simulink model "gm_mandelbrot_fpga"  (R2019b)
settings: Solver=FixedStepDiscrete  StartTime=0.0  StopTime=33.5e-3  FixedStep=0.5*Ts  RelTol=1e-3  EnableMultiTasking=on
undefined symbols (not defined in the file or in its folder): BUTTON_CLOCK_DIV, BUTTON_DEBOUNCE, BUTTON_POLLING, LUT_BLUE, LUT_GREEN, LUT_RED, MAX_ITERATIONS, PIXEL_TIME, TRASLATION_FACTOR, Ts, VGA_HORIZONTAL_BACK_PORCH, VGA_HORIZONTAL_FRONT_PORCH, VGA_HORIZONTAL_RESOLUTION, VGA_HORIZONTAL_SYNC, VGA_VERTICAL_BACK_PORCH, VGA_VERTICAL_FRONT_PORCH, VGA_VERTICAL_RESOLUTION, VGA_VERTICAL_SYNC, ZOOM_FACTOR
libraries: simulink x132, hdlsllib x20, visionsinks x1
(part 3 of 9)

== system gm_mandelbrot_fpga/mandelbrot_top/mandelbrot_core/plane_converter  ==
  zoom : Inport  OutDataTypeStr=fixdt(1, 18, 15)  PortDimensions=1  SampleTime=1.35e-08
  "horizontal_offset " : Inport  Port=2  OutDataTypeStr=fixdt(1, 18, 15)  PortDimensions=1  SampleTime=1.35e-08
  "vertical_offset " : Inport  Port=3  OutDataTypeStr=fixdt(1, 18, 15)  PortDimensions=1  SampleTime=1.35e-08
  "horizontal_index " : Inport  Port=4  OutDataTypeStr=uint16  PortDimensions=1  SampleTime=1.35e-08
  "vertical_index " : Inport  Port=5  OutDataTypeStr=uint16  PortDimensions=1  SampleTime=1.35e-08
  Add : Sum
  Add1 : Sum
  Constant1 : Constant  Value=VGA_VERTICAL_RESOLUTION/2.0  OutDataTypeStr=fixdt(1,12,0)  SampleTime=-1
  Constant2 : Constant  Value=2.0/VGA_VERTICAL_RESOLUTION  OutDataTypeStr=Z_BUS_TYPE  SampleTime=-1
  Constant4 : Constant  Value=VGA_HORIZONTAL_RESOLUTION/2.0  OutDataTypeStr=fixdt(1,12,0)  SampleTime=-1
  Data Type Conversion : DataTypeConversion
  Data Type Conversion1 : DataTypeConversion
  Data Type Conversion2 : DataTypeConversion
  Product1 : Product
  Product2 : Product
  Product3 : Product
  Real-Imag to Complex : RealImagToComplex
  Subtract : Sum  Inputs=-+
  Subtract1 : Sum  Inputs=+-
  Unit Delay : UnitDelay  SampleTime=-1  HasFrameUpgradeWarning=on
  c : Outport  OutDataTypeStr=Z_BUS_TYPE  VectorParamsAs1DForOutWhenUnconnected=off
  wires:
  zoom/1 -> Product1/1
  "horizontal_offset "/1 -> Add/1
  "vertical_offset "/1 -> Add1/1
  "horizontal_index "/1 -> Data Type Conversion/1
  "vertical_index "/1 -> Data Type Conversion1/1
  Add/1 -> Real-Imag to Complex/1
  Add1/1 -> Real-Imag to Complex/2
  Constant1/1 -> Subtract1/1
  Constant2/1 -> Product3/2, Product2/2
  Constant4/1 -> Subtract/1
  Data Type Conversion/1 -> Subtract/2
  Data Type Conversion1/1 -> Subtract1/2
  Data Type Conversion2/1 -> c/1
  Product1/1 -> Data Type Conversion2/1
  Product2/1 -> Add/2
  Product3/1 -> Add1/2
  Real-Imag to Complex/1 -> Unit Delay/1
  Subtract/1 -> Product2/1
  Subtract1/1 -> Product3/1
  Unit Delay/1 -> Product1/2

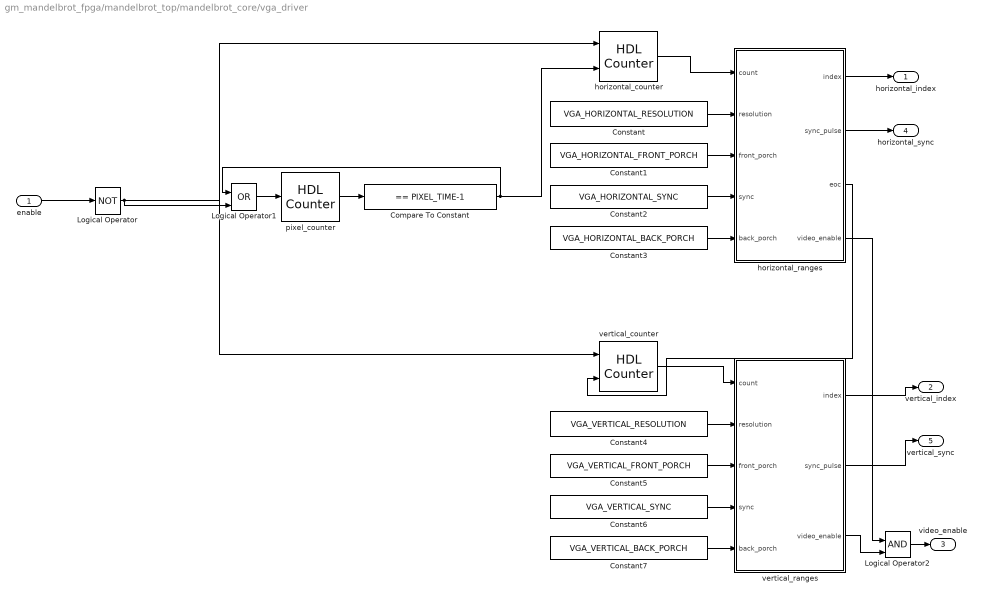
== system gm_mandelbrot_fpga/mandelbrot_top/mandelbrot_core/vga_driver ==
  "enable " : Inport  OutDataTypeStr=boolean  PortDimensions=1  SampleTime=1.35e-08
  Compare To Constant : simulink/Logic and Bit Operations/Compare To Constant  relop===  const=PIXEL_TIME-1  OutDataTypeStr=boolean
  Constant : Constant  Value=VGA_HORIZONTAL_RESOLUTION  OutDataTypeStr=uint16  SampleTime=-1
  Constant1 : Constant  Value=VGA_HORIZONTAL_FRONT_PORCH  OutDataTypeStr=uint16  SampleTime=-1
  Constant2 : Constant  Value=VGA_HORIZONTAL_SYNC  OutDataTypeStr=uint16  SampleTime=-1
  Constant3 : Constant  Value=VGA_HORIZONTAL_BACK_PORCH  OutDataTypeStr=uint16  SampleTime=-1
  Constant4 : Constant  Value=VGA_VERTICAL_RESOLUTION  OutDataTypeStr=uint16  SampleTime=-1
  Constant5 : Constant  Value=VGA_VERTICAL_FRONT_PORCH  OutDataTypeStr=uint16  SampleTime=-1
  Constant6 : Constant  Value=VGA_VERTICAL_SYNC  OutDataTypeStr=uint16  SampleTime=-1
  Constant7 : Constant  Value=VGA_VERTICAL_BACK_PORCH  OutDataTypeStr=uint16  SampleTime=-1
  Logical Operator : Logic  Operator=NOT  IconShape=distinctive  AllPortsSameDT=off  OutDataTypeStr=boolean
  Logical Operator1 : Logic  Operator=OR  IconShape=distinctive  AllPortsSameDT=off  OutDataTypeStr=boolean
  Logical Operator2 : Logic  IconShape=distinctive  AllPortsSameDT=off  OutDataTypeStr=boolean
  horizontal_counter : hdlsllib/Sources/HDL Counter  CountType=Count limited  CountInit=0  CountStep=1  CountMax=VGA_HORIZONTAL_RESOLUTION+VGA_HORIZONTAL_FRONT_PORCH+VGA_HORIZONTAL_SYNC+VGA_HORIZONTAL_BACK_PORCH-1  CountFromType=Initial value  CountFrom=0  CountResetPort=on  CountLoadPort=off  CountEnbPort=on  CountDirPort=off  CountDataType=Unsigned  CountWordLen=16  CountFracLen=0  CountSampTime=1
      settings: SourceProductName=Simulink
  horizontal_ranges : Subsystem
  "pixel_counter " : hdlsllib/Sources/HDL Counter  CountType=Count limited  CountInit=0  CountStep=1  CountMax=PIXEL_TIME  CountFromType=Initial value  CountFrom=0  CountResetPort=on  CountLoadPort=off  CountEnbPort=off  CountDirPort=off  CountDataType=Unsigned  CountWordLen=8  CountFracLen=0  CountSampTime=Ts
      settings: SourceProductName=Simulink
  "vertical_counter " : hdlsllib/Sources/HDL Counter  CountType=Count limited  CountInit=0  CountStep=1  CountMax=VGA_VERTICAL_RESOLUTION+VGA_VERTICAL_FRONT_PORCH+VGA_VERTICAL_SYNC+VGA_VERTICAL_BACK_PORCH-1  CountFromType=Initial value  CountFrom=0  CountResetPort=on  CountLoadPort=off  CountEnbPort=on  CountDirPort=off  CountDataType=Unsigned  CountWordLen=16  CountFracLen=0  CountSampTime=1
      settings: SourceProductName=Simulink
  "vertical_ranges " : Subsystem
  horizontal_index : Outport  VectorParamsAs1DForOutWhenUnconnected=off
  vertical_index : Outport  Port=2  VectorParamsAs1DForOutWhenUnconnected=off
  "video_enable " : Outport  Port=3  OutDataTypeStr=boolean  VectorParamsAs1DForOutWhenUnconnected=off
  horizontal_sync : Outport  Port=4  OutDataTypeStr=boolean  VectorParamsAs1DForOutWhenUnconnected=off
  "vertical_sync " : Outport  Port=5  OutDataTypeStr=boolean  VectorParamsAs1DForOutWhenUnconnected=off
  wires:
  "enable "/1 -> Logical Operator/1
  Compare To Constant/1 -> Logical Operator1/1, horizontal_counter/2
  Constant/1 -> horizontal_ranges/2(resolution)
  Constant1/1 -> horizontal_ranges/3(front_porch)
  Constant2/1 -> horizontal_ranges/4("sync ")
  Constant3/1 -> horizontal_ranges/5(back_porch)
  Constant4/1 -> "vertical_ranges "/2(resolution)
  Constant5/1 -> "vertical_ranges "/3(front_porch)
  Constant6/1 -> "vertical_ranges "/4("sync ")
  Constant7/1 -> "vertical_ranges "/5(back_porch)
  Logical Operator/1 -> Logical Operator1/2, "vertical_counter "/1, horizontal_counter/1
  Logical Operator1/1 -> "pixel_counter "/1
  Logical Operator2/1 -> "video_enable "/1
  horizontal_counter/1 -> horizontal_ranges/1("count ")
  horizontal_ranges/1("index ") -> horizontal_index/1
  horizontal_ranges/2("sync_pulse ") -> horizontal_sync/1
  horizontal_ranges/3("eoc ") -> "vertical_counter "/2
  horizontal_ranges/4(video_enable) -> Logical Operator2/1
  "pixel_counter "/1 -> Compare To Constant/1
  "vertical_counter "/1 -> "vertical_ranges "/1("count ")
  "vertical_ranges "/1("index ") -> vertical_index/1
  "vertical_ranges "/2("sync_pulse ") -> "vertical_sync "/1
  "vertical_ranges "/3(video_enable) -> Logical Operator2/2

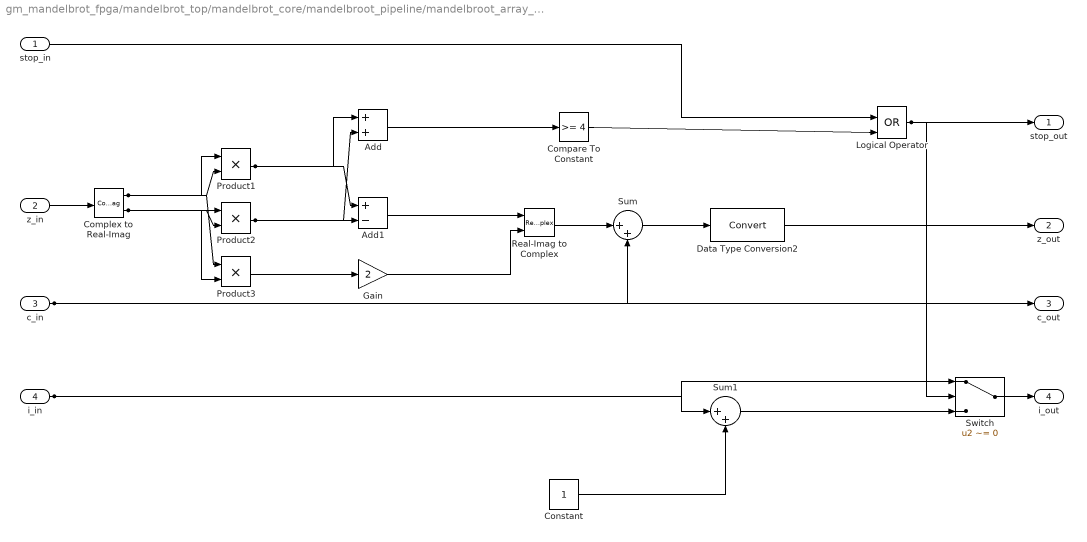
== system gm_mandelbrot_fpga/mandelbrot_top/mandelbrot_core/mandelbroot_pipeline/mandelbroot_array_instance1 ==
  stop_in : Inport  OutDataTypeStr=boolean  PortDimensions=1  SampleTime=1.35e-08
  z_in : Inport  Port=2  OutDataTypeStr=fixdt(1, 18, 15)  PortDimensions=1  SampleTime=1.35e-08
      settings: SignalType=complex
  c_in : Inport  Port=3  OutDataTypeStr=fixdt(1, 18, 15)  PortDimensions=1  SampleTime=1.35e-08
      settings: SignalType=complex
  i_in : Inport  Port=4  OutDataTypeStr=fixdt(0, 7, 0)  PortDimensions=1  SampleTime=1.35e-08
  Add : Sum
  Add1 : Sum  Inputs=+-  OutDataTypeStr=Inherit: Same as first input
  Compare To Constant : simulink/Logic and Bit Operations/Compare To Constant  relop=>=  const=4  OutDataTypeStr=boolean
  Complex to Real-Imag : ComplexToRealImag
  Constant : Constant  OutDataTypeStr=uint8  SampleTime=-1
  Data Type Conversion2 : DataTypeConversion
  Gain : Gain  Gain=2  OutDataTypeStr=Inherit: Same as input  ParamDataTypeStr=Inherit: Same as input
  Logical Operator : Logic  Operator=OR  IconShape=distinctive  AllPortsSameDT=off  OutDataTypeStr=boolean
  Product1 : Product
  Product2 : Product
  Product3 : Product
  Real-Imag to Complex : RealImagToComplex
  Sum : Sum  Inputs=|++  OutDataTypeStr=Inherit: Same as first input
  Sum1 : Sum  Inputs=|++
  Switch : Switch  Criteria=u2 ~= 0
  stop_out : Outport  VectorParamsAs1DForOutWhenUnconnected=off
  z_out : Outport  Port=2  VectorParamsAs1DForOutWhenUnconnected=off
  c_out : Outport  Port=3  VectorParamsAs1DForOutWhenUnconnected=off
  i_out : Outport  Port=4  VectorParamsAs1DForOutWhenUnconnected=off
  wires:
  Switch/1 -> i_out/1
  Sum1/1 -> Switch/3
  Sum/1 -> Data Type Conversion2/1
  Real-Imag to Complex/1 -> Sum/1
  Product3/1 -> Gain/1
  Product2/1 -> Add/2, Add1/2
  Product1/1 -> Add/1, Add1/1
  Logical Operator/1 -> Switch/2, stop_out/1
  Gain/1 -> Real-Imag to Complex/2
  Data Type Conversion2/1 -> z_out/1
  Constant/1 -> Sum1/2
  Complex to Real-Imag/1 -> Product1/2, Product1/1, Product3/1
  Complex to Real-Imag/2 -> Product2/2, Product2/1, Product3/2
  Compare To Constant/1 -> Logical Operator/2
  Add1/1 -> Real-Imag to Complex/1
  Add/1 -> Compare To Constant/1
  stop_in/1 -> Logical Operator/1
  z_in/1 -> Complex to Real-Imag/1
  c_in/1 -> Sum/2, c_out/1
  i_in/1 -> Sum1/1, Switch/1

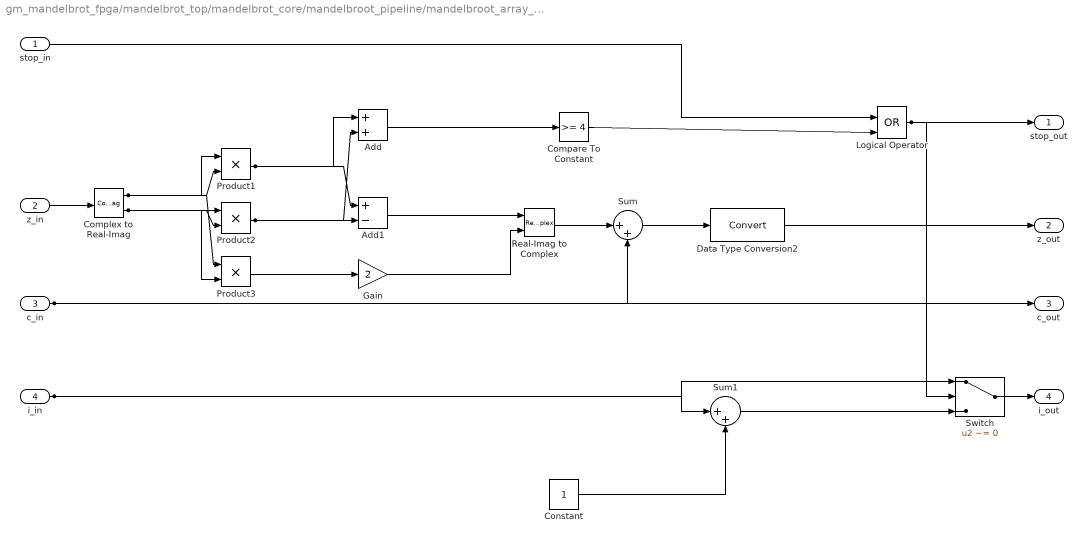
== system gm_mandelbrot_fpga/mandelbrot_top/mandelbrot_core/mandelbroot_pipeline/mandelbroot_array_instance10 ==
  stop_in : Inport  OutDataTypeStr=boolean  PortDimensions=1  SampleTime=1.35e-08
  z_in : Inport  Port=2  OutDataTypeStr=fixdt(1, 18, 15)  PortDimensions=1  SampleTime=1.35e-08
      settings: SignalType=complex
  c_in : Inport  Port=3  OutDataTypeStr=fixdt(1, 18, 15)  PortDimensions=1  SampleTime=1.35e-08
      settings: SignalType=complex
  i_in : Inport  Port=4  OutDataTypeStr=fixdt(0, 7, 0)  PortDimensions=1  SampleTime=1.35e-08
  Add : Sum
  Add1 : Sum  Inputs=+-  OutDataTypeStr=Inherit: Same as first input
  Compare To Constant : simulink/Logic and Bit Operations/Compare To Constant  relop=>=  const=4  OutDataTypeStr=boolean
  Complex to Real-Imag : ComplexToRealImag
  Constant : Constant  OutDataTypeStr=uint8  SampleTime=-1
  Data Type Conversion2 : DataTypeConversion
  Gain : Gain  Gain=2  OutDataTypeStr=Inherit: Same as input  ParamDataTypeStr=Inherit: Same as input
  Logical Operator : Logic  Operator=OR  IconShape=distinctive  AllPortsSameDT=off  OutDataTypeStr=boolean
  Product1 : Product
  Product2 : Product
  Product3 : Product
  Real-Imag to Complex : RealImagToComplex
  Sum : Sum  Inputs=|++  OutDataTypeStr=Inherit: Same as first input
  Sum1 : Sum  Inputs=|++
  Switch : Switch  Criteria=u2 ~= 0
  stop_out : Outport  VectorParamsAs1DForOutWhenUnconnected=off
  z_out : Outport  Port=2  VectorParamsAs1DForOutWhenUnconnected=off
  c_out : Outport  Port=3  VectorParamsAs1DForOutWhenUnconnected=off
  i_out : Outport  Port=4  VectorParamsAs1DForOutWhenUnconnected=off
  wires:
  i_in/1 -> Switch/1, Sum1/1
  c_in/1 -> c_out/1, Sum/2
  z_in/1 -> Complex to Real-Imag/1
  stop_in/1 -> Logical Operator/1
  Add/1 -> Compare To Constant/1
  Add1/1 -> Real-Imag to Complex/1
  Compare To Constant/1 -> Logical Operator/2
  Complex to Real-Imag/2 -> Product3/2, Product2/1, Product2/2
  Complex to Real-Imag/1 -> Product3/1, Product1/1, Product1/2
  Constant/1 -> Sum1/2
  Data Type Conversion2/1 -> z_out/1
  Gain/1 -> Real-Imag to Complex/2
  Logical Operator/1 -> stop_out/1, Switch/2
  Product1/1 -> Add1/1, Add/1
  Product2/1 -> Add1/2, Add/2
  Product3/1 -> Gain/1
  Real-Imag to Complex/1 -> Sum/1
  Sum/1 -> Data Type Conversion2/1
  Sum1/1 -> Switch/3
  Switch/1 -> i_out/1

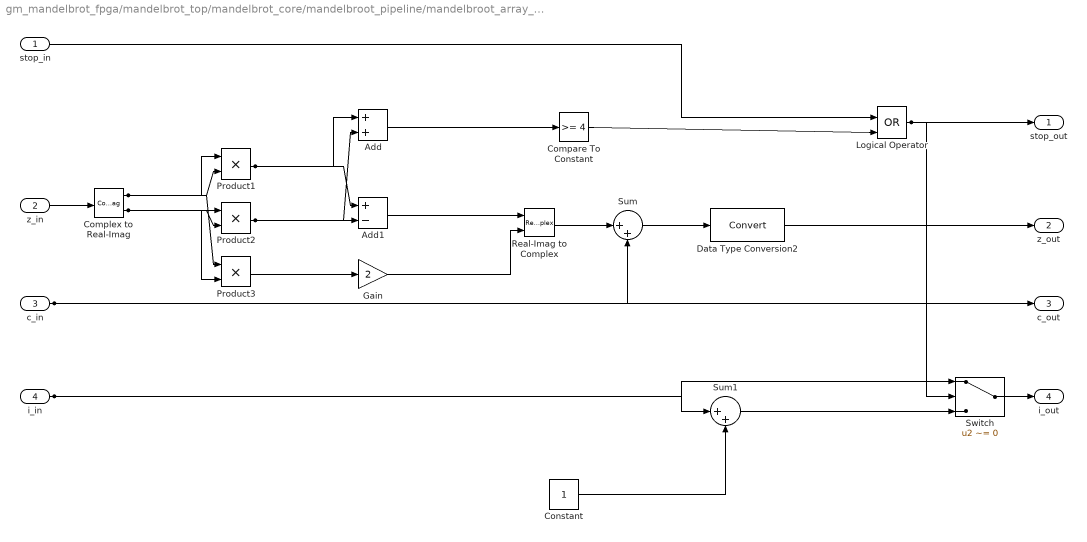
== system gm_mandelbrot_fpga/mandelbrot_top/mandelbrot_core/mandelbroot_pipeline/mandelbroot_array_instance100 ==
  stop_in : Inport  OutDataTypeStr=boolean  PortDimensions=1  SampleTime=1.35e-08
  z_in : Inport  Port=2  OutDataTypeStr=fixdt(1, 18, 15)  PortDimensions=1  SampleTime=1.35e-08
      settings: SignalType=complex
  c_in : Inport  Port=3  OutDataTypeStr=fixdt(1, 18, 15)  PortDimensions=1  SampleTime=1.35e-08
      settings: SignalType=complex
  i_in : Inport  Port=4  OutDataTypeStr=fixdt(0, 7, 0)  PortDimensions=1  SampleTime=1.35e-08
  Add : Sum
  Add1 : Sum  Inputs=+-  OutDataTypeStr=Inherit: Same as first input
  Compare To Constant : simulink/Logic and Bit Operations/Compare To Constant  relop=>=  const=4  OutDataTypeStr=boolean
  Complex to Real-Imag : ComplexToRealImag
  Constant : Constant  OutDataTypeStr=uint8  SampleTime=-1
  Data Type Conversion2 : DataTypeConversion
  Gain : Gain  Gain=2  OutDataTypeStr=Inherit: Same as input  ParamDataTypeStr=Inherit: Same as input
  Logical Operator : Logic  Operator=OR  IconShape=distinctive  AllPortsSameDT=off  OutDataTypeStr=boolean
  Product1 : Product
  Product2 : Product
  Product3 : Product
  Real-Imag to Complex : RealImagToComplex
  Sum : Sum  Inputs=|++  OutDataTypeStr=Inherit: Same as first input
  Sum1 : Sum  Inputs=|++
  Switch : Switch  Criteria=u2 ~= 0
  stop_out : Outport  VectorParamsAs1DForOutWhenUnconnected=off
  z_out : Outport  Port=2  VectorParamsAs1DForOutWhenUnconnected=off
  c_out : Outport  Port=3  VectorParamsAs1DForOutWhenUnconnected=off
  i_out : Outport  Port=4  VectorParamsAs1DForOutWhenUnconnected=off
  wires:
  i_in/1 -> Switch/1, Sum1/1
  c_in/1 -> c_out/1, Sum/2
  z_in/1 -> Complex to Real-Imag/1
  stop_in/1 -> Logical Operator/1
  Add/1 -> Compare To Constant/1
  Add1/1 -> Real-Imag to Complex/1
  Compare To Constant/1 -> Logical Operator/2
  Complex to Real-Imag/2 -> Product3/2, Product2/1, Product2/2
  Complex to Real-Imag/1 -> Product3/1, Product1/1, Product1/2
  Constant/1 -> Sum1/2
  Data Type Conversion2/1 -> z_out/1
  Gain/1 -> Real-Imag to Complex/2
  Logical Operator/1 -> stop_out/1, Switch/2
  Product1/1 -> Add1/1, Add/1
  Product2/1 -> Add1/2, Add/2
  Product3/1 -> Gain/1
  Real-Imag to Complex/1 -> Sum/1
  Sum/1 -> Data Type Conversion2/1
  Sum1/1 -> Switch/3
  Switch/1 -> i_out/1

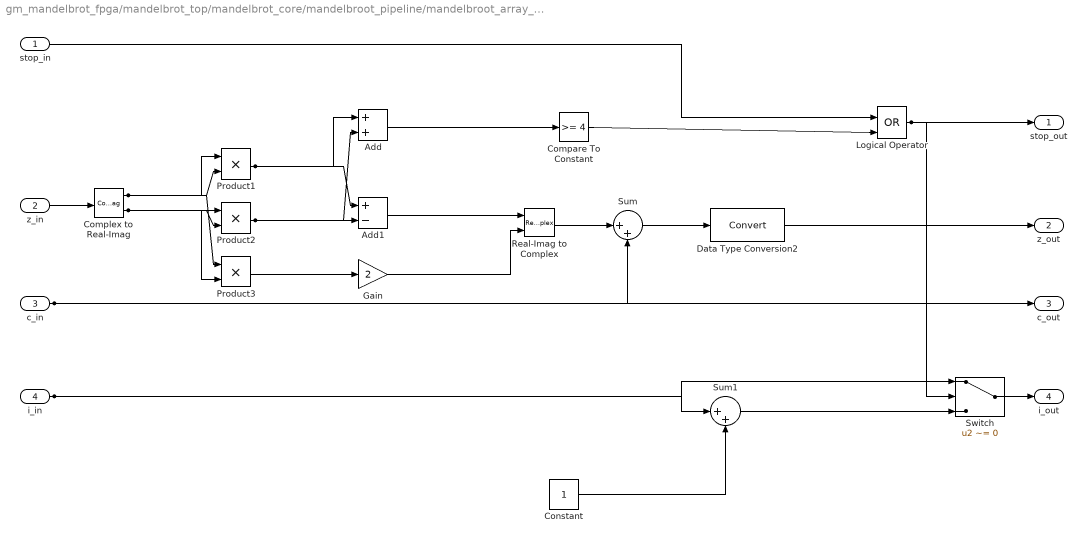
== system gm_mandelbrot_fpga/mandelbrot_top/mandelbrot_core/mandelbroot_pipeline/mandelbroot_array_instance101 ==
  stop_in : Inport  OutDataTypeStr=boolean  PortDimensions=1  SampleTime=1.35e-08
  z_in : Inport  Port=2  OutDataTypeStr=fixdt(1, 18, 15)  PortDimensions=1  SampleTime=1.35e-08
      settings: SignalType=complex
  c_in : Inport  Port=3  OutDataTypeStr=fixdt(1, 18, 15)  PortDimensions=1  SampleTime=1.35e-08
      settings: SignalType=complex
  i_in : Inport  Port=4  OutDataTypeStr=fixdt(0, 7, 0)  PortDimensions=1  SampleTime=1.35e-08
  Add : Sum
  Add1 : Sum  Inputs=+-  OutDataTypeStr=Inherit: Same as first input
  Compare To Constant : simulink/Logic and Bit Operations/Compare To Constant  relop=>=  const=4  OutDataTypeStr=boolean
  Complex to Real-Imag : ComplexToRealImag
  Constant : Constant  OutDataTypeStr=uint8  SampleTime=-1
  Data Type Conversion2 : DataTypeConversion
  Gain : Gain  Gain=2  OutDataTypeStr=Inherit: Same as input  ParamDataTypeStr=Inherit: Same as input
  Logical Operator : Logic  Operator=OR  IconShape=distinctive  AllPortsSameDT=off  OutDataTypeStr=boolean
  Product1 : Product
  Product2 : Product
  Product3 : Product
  Real-Imag to Complex : RealImagToComplex
  Sum : Sum  Inputs=|++  OutDataTypeStr=Inherit: Same as first input
  Sum1 : Sum  Inputs=|++
  Switch : Switch  Criteria=u2 ~= 0
  stop_out : Outport  VectorParamsAs1DForOutWhenUnconnected=off
  z_out : Outport  Port=2  VectorParamsAs1DForOutWhenUnconnected=off
  c_out : Outport  Port=3  VectorParamsAs1DForOutWhenUnconnected=off
  i_out : Outport  Port=4  VectorParamsAs1DForOutWhenUnconnected=off
  wires:
  i_in/1 -> Switch/1, Sum1/1
  c_in/1 -> c_out/1, Sum/2
  z_in/1 -> Complex to Real-Imag/1
  stop_in/1 -> Logical Operator/1
  Add/1 -> Compare To Constant/1
  Add1/1 -> Real-Imag to Complex/1
  Compare To Constant/1 -> Logical Operator/2
  Complex to Real-Imag/2 -> Product3/2, Product2/1, Product2/2
  Complex to Real-Imag/1 -> Product3/1, Product1/1, Product1/2
  Constant/1 -> Sum1/2
  Data Type Conversion2/1 -> z_out/1
  Gain/1 -> Real-Imag to Complex/2
  Logical Operator/1 -> stop_out/1, Switch/2
  Product1/1 -> Add1/1, Add/1
  Product2/1 -> Add1/2, Add/2
  Product3/1 -> Gain/1
  Real-Imag to Complex/1 -> Sum/1
  Sum/1 -> Data Type Conversion2/1
  Sum1/1 -> Switch/3
  Switch/1 -> i_out/1

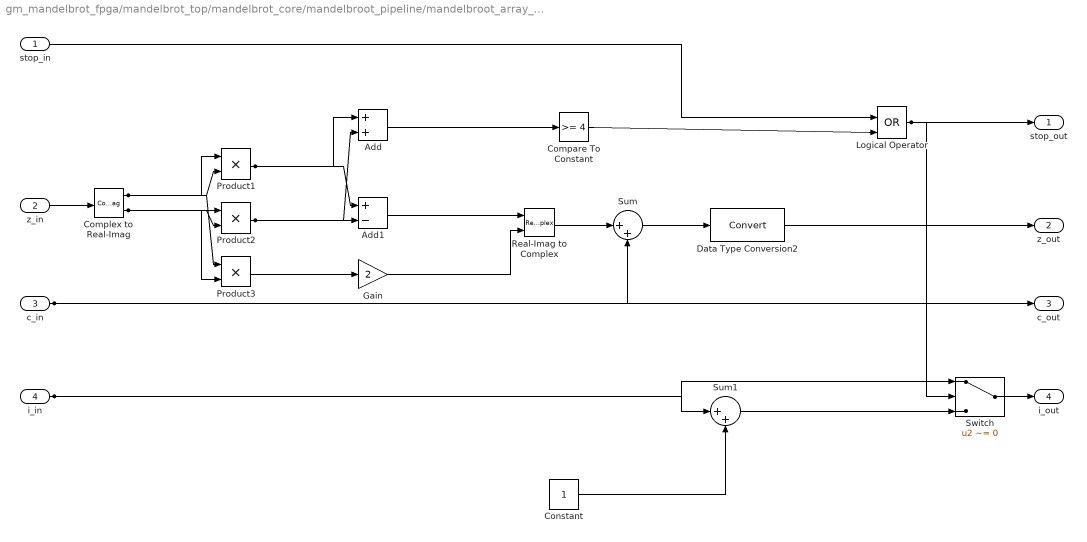
== system gm_mandelbrot_fpga/mandelbrot_top/mandelbrot_core/mandelbroot_pipeline/mandelbroot_array_instance102 ==
  stop_in : Inport  OutDataTypeStr=boolean  PortDimensions=1  SampleTime=1.35e-08
  z_in : Inport  Port=2  OutDataTypeStr=fixdt(1, 18, 15)  PortDimensions=1  SampleTime=1.35e-08
      settings: SignalType=complex
  c_in : Inport  Port=3  OutDataTypeStr=fixdt(1, 18, 15)  PortDimensions=1  SampleTime=1.35e-08
      settings: SignalType=complex
  i_in : Inport  Port=4  OutDataTypeStr=fixdt(0, 7, 0)  PortDimensions=1  SampleTime=1.35e-08
  Add : Sum
  Add1 : Sum  Inputs=+-  OutDataTypeStr=Inherit: Same as first input
  Compare To Constant : simulink/Logic and Bit Operations/Compare To Constant  relop=>=  const=4  OutDataTypeStr=boolean
  Complex to Real-Imag : ComplexToRealImag
  Constant : Constant  OutDataTypeStr=uint8  SampleTime=-1
  Data Type Conversion2 : DataTypeConversion
  Gain : Gain  Gain=2  OutDataTypeStr=Inherit: Same as input  ParamDataTypeStr=Inherit: Same as input
  Logical Operator : Logic  Operator=OR  IconShape=distinctive  AllPortsSameDT=off  OutDataTypeStr=boolean
  Product1 : Product
  Product2 : Product
  Product3 : Product
  Real-Imag to Complex : RealImagToComplex
  Sum : Sum  Inputs=|++  OutDataTypeStr=Inherit: Same as first input
  Sum1 : Sum  Inputs=|++
  Switch : Switch  Criteria=u2 ~= 0
  stop_out : Outport  VectorParamsAs1DForOutWhenUnconnected=off
  z_out : Outport  Port=2  VectorParamsAs1DForOutWhenUnconnected=off
  c_out : Outport  Port=3  VectorParamsAs1DForOutWhenUnconnected=off
  i_out : Outport  Port=4  VectorParamsAs1DForOutWhenUnconnected=off
  wires:
  i_in/1 -> Switch/1, Sum1/1
  c_in/1 -> c_out/1, Sum/2
  z_in/1 -> Complex to Real-Imag/1
  stop_in/1 -> Logical Operator/1
  Add/1 -> Compare To Constant/1
  Add1/1 -> Real-Imag to Complex/1
  Compare To Constant/1 -> Logical Operator/2
  Complex to Real-Imag/2 -> Product3/2, Product2/1, Product2/2
  Complex to Real-Imag/1 -> Product3/1, Product1/1, Product1/2
  Constant/1 -> Sum1/2
  Data Type Conversion2/1 -> z_out/1
  Gain/1 -> Real-Imag to Complex/2
  Logical Operator/1 -> stop_out/1, Switch/2
  Product1/1 -> Add1/1, Add/1
  Product2/1 -> Add1/2, Add/2
  Product3/1 -> Gain/1
  Real-Imag to Complex/1 -> Sum/1
  Sum/1 -> Data Type Conversion2/1
  Sum1/1 -> Switch/3
  Switch/1 -> i_out/1

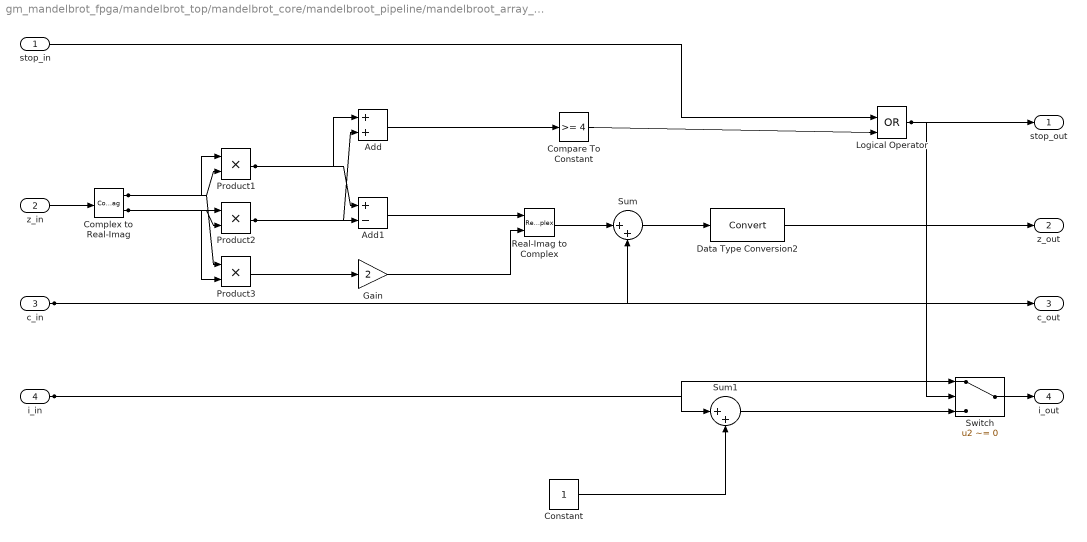
== system gm_mandelbrot_fpga/mandelbrot_top/mandelbrot_core/mandelbroot_pipeline/mandelbroot_array_instance103 ==
  stop_in : Inport  OutDataTypeStr=boolean  PortDimensions=1  SampleTime=1.35e-08
  z_in : Inport  Port=2  OutDataTypeStr=fixdt(1, 18, 15)  PortDimensions=1  SampleTime=1.35e-08
      settings: SignalType=complex
  c_in : Inport  Port=3  OutDataTypeStr=fixdt(1, 18, 15)  PortDimensions=1  SampleTime=1.35e-08
      settings: SignalType=complex
  i_in : Inport  Port=4  OutDataTypeStr=fixdt(0, 7, 0)  PortDimensions=1  SampleTime=1.35e-08
  Add : Sum
  Add1 : Sum  Inputs=+-  OutDataTypeStr=Inherit: Same as first input
  Compare To Constant : simulink/Logic and Bit Operations/Compare To Constant  relop=>=  const=4  OutDataTypeStr=boolean
  Complex to Real-Imag : ComplexToRealImag
  Constant : Constant  OutDataTypeStr=uint8  SampleTime=-1
  Data Type Conversion2 : DataTypeConversion
  Gain : Gain  Gain=2  OutDataTypeStr=Inherit: Same as input  ParamDataTypeStr=Inherit: Same as input
  Logical Operator : Logic  Operator=OR  IconShape=distinctive  AllPortsSameDT=off  OutDataTypeStr=boolean
  Product1 : Product
  Product2 : Product
  Product3 : Product
  Real-Imag to Complex : RealImagToComplex
  Sum : Sum  Inputs=|++  OutDataTypeStr=Inherit: Same as first input
  Sum1 : Sum  Inputs=|++
  Switch : Switch  Criteria=u2 ~= 0
  stop_out : Outport  VectorParamsAs1DForOutWhenUnconnected=off
  z_out : Outport  Port=2  VectorParamsAs1DForOutWhenUnconnected=off
  c_out : Outport  Port=3  VectorParamsAs1DForOutWhenUnconnected=off
  i_out : Outport  Port=4  VectorParamsAs1DForOutWhenUnconnected=off
  wires:
  i_in/1 -> Switch/1, Sum1/1
  c_in/1 -> c_out/1, Sum/2
  z_in/1 -> Complex to Real-Imag/1
  stop_in/1 -> Logical Operator/1
  Add/1 -> Compare To Constant/1
  Add1/1 -> Real-Imag to Complex/1
  Compare To Constant/1 -> Logical Operator/2
  Complex to Real-Imag/2 -> Product3/2, Product2/1, Product2/2
  Complex to Real-Imag/1 -> Product3/1, Product1/1, Product1/2
  Constant/1 -> Sum1/2
  Data Type Conversion2/1 -> z_out/1
  Gain/1 -> Real-Imag to Complex/2
  Logical Operator/1 -> stop_out/1, Switch/2
  Product1/1 -> Add1/1, Add/1
  Product2/1 -> Add1/2, Add/2
  Product3/1 -> Gain/1
  Real-Imag to Complex/1 -> Sum/1
  Sum/1 -> Data Type Conversion2/1
  Sum1/1 -> Switch/3
  Switch/1 -> i_out/1

== system gm_mandelbrot_fpga/mandelbrot_top/mandelbrot_core/mandelbroot_pipeline/mandelbroot_array_instance104 ==
  stop_in : Inport  OutDataTypeStr=boolean  PortDimensions=1  SampleTime=1.35e-08
  z_in : Inport  Port=2  OutDataTypeStr=fixdt(1, 18, 15)  PortDimensions=1  SampleTime=1.35e-08
      settings: SignalType=complex
  c_in : Inport  Port=3  OutDataTypeStr=fixdt(1, 18, 15)  PortDimensions=1  SampleTime=1.35e-08
      settings: SignalType=complex
  i_in : Inport  Port=4  OutDataTypeStr=fixdt(0, 7, 0)  PortDimensions=1  SampleTime=1.35e-08
  Add : Sum
  Add1 : Sum  Inputs=+-  OutDataTypeStr=Inherit: Same as first input
  Compare To Constant : simulink/Logic and Bit Operations/Compare To Constant  relop=>=  const=4  OutDataTypeStr=boolean
  Complex to Real-Imag : ComplexToRealImag
  Constant : Constant  OutDataTypeStr=uint8  SampleTime=-1
  Data Type Conversion2 : DataTypeConversion
  Gain : Gain  Gain=2  OutDataTypeStr=Inherit: Same as input  ParamDataTypeStr=Inherit: Same as input
  Logical Operator : Logic  Operator=OR  IconShape=distinctive  AllPortsSameDT=off  OutDataTypeStr=boolean
  Product1 : Product
  Product2 : Product
  Product3 : Product
  Real-Imag to Complex : RealImagToComplex
  Sum : Sum  Inputs=|++  OutDataTypeStr=Inherit: Same as first input
  Sum1 : Sum  Inputs=|++
  Switch : Switch  Criteria=u2 ~= 0
  stop_out : Outport  VectorParamsAs1DForOutWhenUnconnected=off
  z_out : Outport  Port=2  VectorParamsAs1DForOutWhenUnconnected=off
  c_out : Outport  Port=3  VectorParamsAs1DForOutWhenUnconnected=off
  i_out : Outport  Port=4  VectorParamsAs1DForOutWhenUnconnected=off
  wires:
  i_in/1 -> Switch/1, Sum1/1
  c_in/1 -> c_out/1, Sum/2
  z_in/1 -> Complex to Real-Imag/1
  stop_in/1 -> Logical Operator/1
  Add/1 -> Compare To Constant/1
  Add1/1 -> Real-Imag to Complex/1
  Compare To Constant/1 -> Logical Operator/2
  Complex to Real-Imag/2 -> Product3/2, Product2/1, Product2/2
  Complex to Real-Imag/1 -> Product3/1, Product1/1, Product1/2
  Constant/1 -> Sum1/2
  Data Type Conversion2/1 -> z_out/1
  Gain/1 -> Real-Imag to Complex/2
  Logical Operator/1 -> stop_out/1, Switch/2
  Product1/1 -> Add1/1, Add/1
  Product2/1 -> Add1/2, Add/2
  Product3/1 -> Gain/1
  Real-Imag to Complex/1 -> Sum/1
  Sum/1 -> Data Type Conversion2/1
  Sum1/1 -> Switch/3
  Switch/1 -> i_out/1

== system gm_mandelbrot_fpga/mandelbrot_top/mandelbrot_core/mandelbroot_pipeline/mandelbroot_array_instance105 ==
  stop_in : Inport  OutDataTypeStr=boolean  PortDimensions=1  SampleTime=1.35e-08
  z_in : Inport  Port=2  OutDataTypeStr=fixdt(1, 18, 15)  PortDimensions=1  SampleTime=1.35e-08
      settings: SignalType=complex
  c_in : Inport  Port=3  OutDataTypeStr=fixdt(1, 18, 15)  PortDimensions=1  SampleTime=1.35e-08
      settings: SignalType=complex
  i_in : Inport  Port=4  OutDataTypeStr=fixdt(0, 7, 0)  PortDimensions=1  SampleTime=1.35e-08
  Add : Sum
  Add1 : Sum  Inputs=+-  OutDataTypeStr=Inherit: Same as first input
  Compare To Constant : simulink/Logic and Bit Operations/Compare To Constant  relop=>=  const=4  OutDataTypeStr=boolean
  Complex to Real-Imag : ComplexToRealImag
  Constant : Constant  OutDataTypeStr=uint8  SampleTime=-1
  Data Type Conversion2 : DataTypeConversion
  Gain : Gain  Gain=2  OutDataTypeStr=Inherit: Same as input  ParamDataTypeStr=Inherit: Same as input
  Logical Operator : Logic  Operator=OR  IconShape=distinctive  AllPortsSameDT=off  OutDataTypeStr=boolean
  Product1 : Product
  Product2 : Product
  Product3 : Product
  Real-Imag to Complex : RealImagToComplex
  Sum : Sum  Inputs=|++  OutDataTypeStr=Inherit: Same as first input
  Sum1 : Sum  Inputs=|++
  Switch : Switch  Criteria=u2 ~= 0
  stop_out : Outport  VectorParamsAs1DForOutWhenUnconnected=off
  z_out : Outport  Port=2  VectorParamsAs1DForOutWhenUnconnected=off
  c_out : Outport  Port=3  VectorParamsAs1DForOutWhenUnconnected=off
  i_out : Outport  Port=4  VectorParamsAs1DForOutWhenUnconnected=off
  wires:
  i_in/1 -> Switch/1, Sum1/1
  c_in/1 -> c_out/1, Sum/2
  z_in/1 -> Complex to Real-Imag/1
  stop_in/1 -> Logical Operator/1
  Add/1 -> Compare To Constant/1
  Add1/1 -> Real-Imag to Complex/1
  Compare To Constant/1 -> Logical Operator/2
  Complex to Real-Imag/2 -> Product3/2, Product2/1, Product2/2
  Complex to Real-Imag/1 -> Product3/1, Product1/1, Product1/2
  Constant/1 -> Sum1/2
  Data Type Conversion2/1 -> z_out/1
  Gain/1 -> Real-Imag to Complex/2
  Logical Operator/1 -> stop_out/1, Switch/2
  Product1/1 -> Add1/1, Add/1
  Product2/1 -> Add1/2, Add/2
  Product3/1 -> Gain/1
  Real-Imag to Complex/1 -> Sum/1
  Sum/1 -> Data Type Conversion2/1
  Sum1/1 -> Switch/3
  Switch/1 -> i_out/1

== system gm_mandelbrot_fpga/mandelbrot_top/mandelbrot_core/mandelbroot_pipeline/mandelbroot_array_instance106 ==
  stop_in : Inport  OutDataTypeStr=boolean  PortDimensions=1  SampleTime=1.35e-08
  z_in : Inport  Port=2  OutDataTypeStr=fixdt(1, 18, 15)  PortDimensions=1  SampleTime=1.35e-08
      settings: SignalType=complex
  c_in : Inport  Port=3  OutDataTypeStr=fixdt(1, 18, 15)  PortDimensions=1  SampleTime=1.35e-08
      settings: SignalType=complex
  i_in : Inport  Port=4  OutDataTypeStr=fixdt(0, 7, 0)  PortDimensions=1  SampleTime=1.35e-08
  Add : Sum
  Add1 : Sum  Inputs=+-  OutDataTypeStr=Inherit: Same as first input
  Compare To Constant : simulink/Logic and Bit Operations/Compare To Constant  relop=>=  const=4  OutDataTypeStr=boolean
  Complex to Real-Imag : ComplexToRealImag
  Constant : Constant  OutDataTypeStr=uint8  SampleTime=-1
  Data Type Conversion2 : DataTypeConversion
  Gain : Gain  Gain=2  OutDataTypeStr=Inherit: Same as input  ParamDataTypeStr=Inherit: Same as input
  Logical Operator : Logic  Operator=OR  IconShape=distinctive  AllPortsSameDT=off  OutDataTypeStr=boolean
  Product1 : Product
  Product2 : Product
  Product3 : Product
  Real-Imag to Complex : RealImagToComplex
  Sum : Sum  Inputs=|++  OutDataTypeStr=Inherit: Same as first input
  Sum1 : Sum  Inputs=|++
  Switch : Switch  Criteria=u2 ~= 0
  stop_out : Outport  VectorParamsAs1DForOutWhenUnconnected=off
  z_out : Outport  Port=2  VectorParamsAs1DForOutWhenUnconnected=off
  c_out : Outport  Port=3  VectorParamsAs1DForOutWhenUnconnected=off
  i_out : Outport  Port=4  VectorParamsAs1DForOutWhenUnconnected=off
  wires:
  i_in/1 -> Switch/1, Sum1/1
  c_in/1 -> c_out/1, Sum/2
  z_in/1 -> Complex to Real-Imag/1
  stop_in/1 -> Logical Operator/1
  Add/1 -> Compare To Constant/1
  Add1/1 -> Real-Imag to Complex/1
  Compare To Constant/1 -> Logical Operator/2
  Complex to Real-Imag/2 -> Product3/2, Product2/1, Product2/2
  Complex to Real-Imag/1 -> Product3/1, Product1/1, Product1/2
  Constant/1 -> Sum1/2
  Data Type Conversion2/1 -> z_out/1
  Gain/1 -> Real-Imag to Complex/2
  Logical Operator/1 -> stop_out/1, Switch/2
  Product1/1 -> Add1/1, Add/1
  Product2/1 -> Add1/2, Add/2
  Product3/1 -> Gain/1
  Real-Imag to Complex/1 -> Sum/1
  Sum/1 -> Data Type Conversion2/1
  Sum1/1 -> Switch/3
  Switch/1 -> i_out/1

== system gm_mandelbrot_fpga/mandelbrot_top/mandelbrot_core/mandelbroot_pipeline/mandelbroot_array_instance107 ==
  stop_in : Inport  OutDataTypeStr=boolean  PortDimensions=1  SampleTime=1.35e-08
  z_in : Inport  Port=2  OutDataTypeStr=fixdt(1, 18, 15)  PortDimensions=1  SampleTime=1.35e-08
      settings: SignalType=complex
  c_in : Inport  Port=3  OutDataTypeStr=fixdt(1, 18, 15)  PortDimensions=1  SampleTime=1.35e-08
      settings: SignalType=complex
  i_in : Inport  Port=4  OutDataTypeStr=fixdt(0, 7, 0)  PortDimensions=1  SampleTime=1.35e-08
  Add : Sum
  Add1 : Sum  Inputs=+-  OutDataTypeStr=Inherit: Same as first input
  Compare To Constant : simulink/Logic and Bit Operations/Compare To Constant  relop=>=  const=4  OutDataTypeStr=boolean
  Complex to Real-Imag : ComplexToRealImag
  Constant : Constant  OutDataTypeStr=uint8  SampleTime=-1
  Data Type Conversion2 : DataTypeConversion
  Gain : Gain  Gain=2  OutDataTypeStr=Inherit: Same as input  ParamDataTypeStr=Inherit: Same as input
  Logical Operator : Logic  Operator=OR  IconShape=distinctive  AllPortsSameDT=off  OutDataTypeStr=boolean
  Product1 : Product
  Product2 : Product
  Product3 : Product
  Real-Imag to Complex : RealImagToComplex
  Sum : Sum  Inputs=|++  OutDataTypeStr=Inherit: Same as first input
  Sum1 : Sum  Inputs=|++
  Switch : Switch  Criteria=u2 ~= 0
  stop_out : Outport  VectorParamsAs1DForOutWhenUnconnected=off
  z_out : Outport  Port=2  VectorParamsAs1DForOutWhenUnconnected=off
  c_out : Outport  Port=3  VectorParamsAs1DForOutWhenUnconnected=off
  i_out : Outport  Port=4  VectorParamsAs1DForOutWhenUnconnected=off
  wires:
  i_in/1 -> Switch/1, Sum1/1
  c_in/1 -> c_out/1, Sum/2
  z_in/1 -> Complex to Real-Imag/1
  stop_in/1 -> Logical Operator/1
  Add/1 -> Compare To Constant/1
  Add1/1 -> Real-Imag to Complex/1
  Compare To Constant/1 -> Logical Operator/2
  Complex to Real-Imag/2 -> Product3/2, Product2/1, Product2/2
  Complex to Real-Imag/1 -> Product3/1, Product1/1, Product1/2
  Constant/1 -> Sum1/2
  Data Type Conversion2/1 -> z_out/1
  Gain/1 -> Real-Imag to Complex/2
  Logical Operator/1 -> stop_out/1, Switch/2
  Product1/1 -> Add1/1, Add/1
  Product2/1 -> Add1/2, Add/2
  Product3/1 -> Gain/1
  Real-Imag to Complex/1 -> Sum/1
  Sum/1 -> Data Type Conversion2/1
  Sum1/1 -> Switch/3
  Switch/1 -> i_out/1

== system gm_mandelbrot_fpga/mandelbrot_top/mandelbrot_core/mandelbroot_pipeline/mandelbroot_array_instance108 ==
  stop_in : Inport  OutDataTypeStr=boolean  PortDimensions=1  SampleTime=1.35e-08
  z_in : Inport  Port=2  OutDataTypeStr=fixdt(1, 18, 15)  PortDimensions=1  SampleTime=1.35e-08
      settings: SignalType=complex
  c_in : Inport  Port=3  OutDataTypeStr=fixdt(1, 18, 15)  PortDimensions=1  SampleTime=1.35e-08
      settings: SignalType=complex
  i_in : Inport  Port=4  OutDataTypeStr=fixdt(0, 7, 0)  PortDimensions=1  SampleTime=1.35e-08
  Add : Sum
  Add1 : Sum  Inputs=+-  OutDataTypeStr=Inherit: Same as first input
  Compare To Constant : simulink/Logic and Bit Operations/Compare To Constant  relop=>=  const=4  OutDataTypeStr=boolean
  Complex to Real-Imag : ComplexToRealImag
  Constant : Constant  OutDataTypeStr=uint8  SampleTime=-1
  Data Type Conversion2 : DataTypeConversion
  Gain : Gain  Gain=2  OutDataTypeStr=Inherit: Same as input  ParamDataTypeStr=Inherit: Same as input
  Logical Operator : Logic  Operator=OR  IconShape=distinctive  AllPortsSameDT=off  OutDataTypeStr=boolean
  Product1 : Product
  Product2 : Product
  Product3 : Product
  Real-Imag to Complex : RealImagToComplex
  Sum : Sum  Inputs=|++  OutDataTypeStr=Inherit: Same as first input
  Sum1 : Sum  Inputs=|++
  Switch : Switch  Criteria=u2 ~= 0
  stop_out : Outport  VectorParamsAs1DForOutWhenUnconnected=off
  z_out : Outport  Port=2  VectorParamsAs1DForOutWhenUnconnected=off
  c_out : Outport  Port=3  VectorParamsAs1DForOutWhenUnconnected=off
  i_out : Outport  Port=4  VectorParamsAs1DForOutWhenUnconnected=off
  wires:
  i_in/1 -> Switch/1, Sum1/1
  c_in/1 -> c_out/1, Sum/2
  z_in/1 -> Complex to Real-Imag/1
  stop_in/1 -> Logical Operator/1
  Add/1 -> Compare To Constant/1
  Add1/1 -> Real-Imag to Complex/1
  Compare To Constant/1 -> Logical Operator/2
  Complex to Real-Imag/2 -> Product3/2, Product2/1, Product2/2
  Complex to Real-Imag/1 -> Product3/1, Product1/1, Product1/2
  Constant/1 -> Sum1/2
  Data Type Conversion2/1 -> z_out/1
  Gain/1 -> Real-Imag to Complex/2
  Logical Operator/1 -> stop_out/1, Switch/2
  Product1/1 -> Add1/1, Add/1
  Product2/1 -> Add1/2, Add/2
  Product3/1 -> Gain/1
  Real-Imag to Complex/1 -> Sum/1
  Sum/1 -> Data Type Conversion2/1
  Sum1/1 -> Switch/3
  Switch/1 -> i_out/1

== system gm_mandelbrot_fpga/mandelbrot_top/mandelbrot_core/mandelbroot_pipeline/mandelbroot_array_instance109 ==
  stop_in : Inport  OutDataTypeStr=boolean  PortDimensions=1  SampleTime=1.35e-08
  z_in : Inport  Port=2  OutDataTypeStr=fixdt(1, 18, 15)  PortDimensions=1  SampleTime=1.35e-08
      settings: SignalType=complex
  c_in : Inport  Port=3  OutDataTypeStr=fixdt(1, 18, 15)  PortDimensions=1  SampleTime=1.35e-08
      settings: SignalType=complex
  i_in : Inport  Port=4  OutDataTypeStr=fixdt(0, 7, 0)  PortDimensions=1  SampleTime=1.35e-08
  Add : Sum
  Add1 : Sum  Inputs=+-  OutDataTypeStr=Inherit: Same as first input
  Compare To Constant : simulink/Logic and Bit Operations/Compare To Constant  relop=>=  const=4  OutDataTypeStr=boolean
  Complex to Real-Imag : ComplexToRealImag
  Constant : Constant  OutDataTypeStr=uint8  SampleTime=-1
  Data Type Conversion2 : DataTypeConversion
  Gain : Gain  Gain=2  OutDataTypeStr=Inherit: Same as input  ParamDataTypeStr=Inherit: Same as input
  Logical Operator : Logic  Operator=OR  IconShape=distinctive  AllPortsSameDT=off  OutDataTypeStr=boolean
  Product1 : Product
  Product2 : Product
  Product3 : Product
  Real-Imag to Complex : RealImagToComplex
  Sum : Sum  Inputs=|++  OutDataTypeStr=Inherit: Same as first input
  Sum1 : Sum  Inputs=|++
  Switch : Switch  Criteria=u2 ~= 0
  stop_out : Outport  VectorParamsAs1DForOutWhenUnconnected=off
  z_out : Outport  Port=2  VectorParamsAs1DForOutWhenUnconnected=off
  c_out : Outport  Port=3  VectorParamsAs1DForOutWhenUnconnected=off
  i_out : Outport  Port=4  VectorParamsAs1DForOutWhenUnconnected=off
  wires:
  i_in/1 -> Switch/1, Sum1/1
  c_in/1 -> c_out/1, Sum/2
  z_in/1 -> Complex to Real-Imag/1
  stop_in/1 -> Logical Operator/1
  Add/1 -> Compare To Constant/1
  Add1/1 -> Real-Imag to Complex/1
  Compare To Constant/1 -> Logical Operator/2
  Complex to Real-Imag/2 -> Product3/2, Product2/1, Product2/2
  Complex to Real-Imag/1 -> Product3/1, Product1/1, Product1/2
  Constant/1 -> Sum1/2
  Data Type Conversion2/1 -> z_out/1
  Gain/1 -> Real-Imag to Complex/2
  Logical Operator/1 -> stop_out/1, Switch/2
  Product1/1 -> Add1/1, Add/1
  Product2/1 -> Add1/2, Add/2
  Product3/1 -> Gain/1
  Real-Imag to Complex/1 -> Sum/1
  Sum/1 -> Data Type Conversion2/1
  Sum1/1 -> Switch/3
  Switch/1 -> i_out/1

== system gm_mandelbrot_fpga/mandelbrot_top/mandelbrot_core/mandelbroot_pipeline/mandelbroot_array_instance11 ==
  stop_in : Inport  OutDataTypeStr=boolean  PortDimensions=1  SampleTime=1.35e-08
  z_in : Inport  Port=2  OutDataTypeStr=fixdt(1, 18, 15)  PortDimensions=1  SampleTime=1.35e-08
      settings: SignalType=complex
  c_in : Inport  Port=3  OutDataTypeStr=fixdt(1, 18, 15)  PortDimensions=1  SampleTime=1.35e-08
      settings: SignalType=complex
  i_in : Inport  Port=4  OutDataTypeStr=fixdt(0, 7, 0)  PortDimensions=1  SampleTime=1.35e-08
  Add : Sum
  Add1 : Sum  Inputs=+-  OutDataTypeStr=Inherit: Same as first input
  Compare To Constant : simulink/Logic and Bit Operations/Compare To Constant  relop=>=  const=4  OutDataTypeStr=boolean
  Complex to Real-Imag : ComplexToRealImag
  Constant : Constant  OutDataTypeStr=uint8  SampleTime=-1
  Data Type Conversion2 : DataTypeConversion
  Gain : Gain  Gain=2  OutDataTypeStr=Inherit: Same as input  ParamDataTypeStr=Inherit: Same as input
  Logical Operator : Logic  Operator=OR  IconShape=distinctive  AllPortsSameDT=off  OutDataTypeStr=boolean
  Product1 : Product
  Product2 : Product
  Product3 : Product
  Real-Imag to Complex : RealImagToComplex
  Sum : Sum  Inputs=|++  OutDataTypeStr=Inherit: Same as first input
  Sum1 : Sum  Inputs=|++
  Switch : Switch  Criteria=u2 ~= 0
  stop_out : Outport  VectorParamsAs1DForOutWhenUnconnected=off
  z_out : Outport  Port=2  VectorParamsAs1DForOutWhenUnconnected=off
  c_out : Outport  Port=3  VectorParamsAs1DForOutWhenUnconnected=off
  i_out : Outport  Port=4  VectorParamsAs1DForOutWhenUnconnected=off
  wires:
  i_in/1 -> Switch/1, Sum1/1
  c_in/1 -> c_out/1, Sum/2
  z_in/1 -> Complex to Real-Imag/1
  stop_in/1 -> Logical Operator/1
  Add/1 -> Compare To Constant/1
  Add1/1 -> Real-Imag to Complex/1
  Compare To Constant/1 -> Logical Operator/2
  Complex to Real-Imag/2 -> Product3/2, Product2/1, Product2/2
  Complex to Real-Imag/1 -> Product3/1, Product1/1, Product1/2
  Constant/1 -> Sum1/2
  Data Type Conversion2/1 -> z_out/1
  Gain/1 -> Real-Imag to Complex/2
  Logical Operator/1 -> stop_out/1, Switch/2
  Product1/1 -> Add1/1, Add/1
  Product2/1 -> Add1/2, Add/2
  Product3/1 -> Gain/1
  Real-Imag to Complex/1 -> Sum/1
  Sum/1 -> Data Type Conversion2/1
  Sum1/1 -> Switch/3
  Switch/1 -> i_out/1

== system gm_mandelbrot_fpga/mandelbrot_top/mandelbrot_core/mandelbroot_pipeline/mandelbroot_array_instance110 ==
  stop_in : Inport  OutDataTypeStr=boolean  PortDimensions=1  SampleTime=1.35e-08
  z_in : Inport  Port=2  OutDataTypeStr=fixdt(1, 18, 15)  PortDimensions=1  SampleTime=1.35e-08
      settings: SignalType=complex
  c_in : Inport  Port=3  OutDataTypeStr=fixdt(1, 18, 15)  PortDimensions=1  SampleTime=1.35e-08
      settings: SignalType=complex
  i_in : Inport  Port=4  OutDataTypeStr=fixdt(0, 7, 0)  PortDimensions=1  SampleTime=1.35e-08
  Add : Sum
  Add1 : Sum  Inputs=+-  OutDataTypeStr=Inherit: Same as first input
  Compare To Constant : simulink/Logic and Bit Operations/Compare To Constant  relop=>=  const=4  OutDataTypeStr=boolean
  Complex to Real-Imag : ComplexToRealImag
  Constant : Constant  OutDataTypeStr=uint8  SampleTime=-1
  Data Type Conversion2 : DataTypeConversion
  Gain : Gain  Gain=2  OutDataTypeStr=Inherit: Same as input  ParamDataTypeStr=Inherit: Same as input
  Logical Operator : Logic  Operator=OR  IconShape=distinctive  AllPortsSameDT=off  OutDataTypeStr=boolean
  Product1 : Product
  Product2 : Product
  Product3 : Product
  Real-Imag to Complex : RealImagToComplex
  Sum : Sum  Inputs=|++  OutDataTypeStr=Inherit: Same as first input
  Sum1 : Sum  Inputs=|++
  Switch : Switch  Criteria=u2 ~= 0
  stop_out : Outport  VectorParamsAs1DForOutWhenUnconnected=off
  z_out : Outport  Port=2  VectorParamsAs1DForOutWhenUnconnected=off
  c_out : Outport  Port=3  VectorParamsAs1DForOutWhenUnconnected=off
  i_out : Outport  Port=4  VectorParamsAs1DForOutWhenUnconnected=off
  wires:
  i_in/1 -> Switch/1, Sum1/1
  c_in/1 -> c_out/1, Sum/2
  z_in/1 -> Complex to Real-Imag/1
  stop_in/1 -> Logical Operator/1
  Add/1 -> Compare To Constant/1
  Add1/1 -> Real-Imag to Complex/1
  Compare To Constant/1 -> Logical Operator/2
  Complex to Real-Imag/2 -> Product3/2, Product2/1, Product2/2
  Complex to Real-Imag/1 -> Product3/1, Product1/1, Product1/2
  Constant/1 -> Sum1/2
  Data Type Conversion2/1 -> z_out/1
  Gain/1 -> Real-Imag to Complex/2
  Logical Operator/1 -> stop_out/1, Switch/2
  Product1/1 -> Add1/1, Add/1
  Product2/1 -> Add1/2, Add/2
  Product3/1 -> Gain/1
  Real-Imag to Complex/1 -> Sum/1
  Sum/1 -> Data Type Conversion2/1
  Sum1/1 -> Switch/3
  Switch/1 -> i_out/1

== system gm_mandelbrot_fpga/mandelbrot_top/mandelbrot_core/mandelbroot_pipeline/mandelbroot_array_instance111 ==
  stop_in : Inport  OutDataTypeStr=boolean  PortDimensions=1  SampleTime=1.35e-08
  z_in : Inport  Port=2  OutDataTypeStr=fixdt(1, 18, 15)  PortDimensions=1  SampleTime=1.35e-08
      settings: SignalType=complex
  c_in : Inport  Port=3  OutDataTypeStr=fixdt(1, 18, 15)  PortDimensions=1  SampleTime=1.35e-08
      settings: SignalType=complex
  i_in : Inport  Port=4  OutDataTypeStr=fixdt(0, 7, 0)  PortDimensions=1  SampleTime=1.35e-08
  Add : Sum
  Add1 : Sum  Inputs=+-  OutDataTypeStr=Inherit: Same as first input
  Compare To Constant : simulink/Logic and Bit Operations/Compare To Constant  relop=>=  const=4  OutDataTypeStr=boolean
  Complex to Real-Imag : ComplexToRealImag
  Constant : Constant  OutDataTypeStr=uint8  SampleTime=-1
  Data Type Conversion2 : DataTypeConversion
  Gain : Gain  Gain=2  OutDataTypeStr=Inherit: Same as input  ParamDataTypeStr=Inherit: Same as input
  Logical Operator : Logic  Operator=OR  IconShape=distinctive  AllPortsSameDT=off  OutDataTypeStr=boolean
  Product1 : Product
  Product2 : Product
  Product3 : Product
  Real-Imag to Complex : RealImagToComplex
  Sum : Sum  Inputs=|++  OutDataTypeStr=Inherit: Same as first input
  Sum1 : Sum  Inputs=|++
  Switch : Switch  Criteria=u2 ~= 0
  stop_out : Outport  VectorParamsAs1DForOutWhenUnconnected=off
  z_out : Outport  Port=2  VectorParamsAs1DForOutWhenUnconnected=off
  c_out : Outport  Port=3  VectorParamsAs1DForOutWhenUnconnected=off
  i_out : Outport  Port=4  VectorParamsAs1DForOutWhenUnconnected=off
  wires:
  i_in/1 -> Switch/1, Sum1/1
  c_in/1 -> c_out/1, Sum/2
  z_in/1 -> Complex to Real-Imag/1
  stop_in/1 -> Logical Operator/1
  Add/1 -> Compare To Constant/1
  Add1/1 -> Real-Imag to Complex/1
  Compare To Constant/1 -> Logical Operator/2
  Complex to Real-Imag/2 -> Product3/2, Product2/1, Product2/2
  Complex to Real-Imag/1 -> Product3/1, Product1/1, Product1/2
  Constant/1 -> Sum1/2
  Data Type Conversion2/1 -> z_out/1
  Gain/1 -> Real-Imag to Complex/2
  Logical Operator/1 -> stop_out/1, Switch/2
  Product1/1 -> Add1/1, Add/1
  Product2/1 -> Add1/2, Add/2
  Product3/1 -> Gain/1
  Real-Imag to Complex/1 -> Sum/1
  Sum/1 -> Data Type Conversion2/1
  Sum1/1 -> Switch/3
  Switch/1 -> i_out/1

== system gm_mandelbrot_fpga/mandelbrot_top/mandelbrot_core/mandelbroot_pipeline/mandelbroot_array_instance112 ==
  stop_in : Inport  OutDataTypeStr=boolean  PortDimensions=1  SampleTime=1.35e-08
  z_in : Inport  Port=2  OutDataTypeStr=fixdt(1, 18, 15)  PortDimensions=1  SampleTime=1.35e-08
      settings: SignalType=complex
  c_in : Inport  Port=3  OutDataTypeStr=fixdt(1, 18, 15)  PortDimensions=1  SampleTime=1.35e-08
      settings: SignalType=complex
  i_in : Inport  Port=4  OutDataTypeStr=fixdt(0, 7, 0)  PortDimensions=1  SampleTime=1.35e-08
  Add : Sum
  Add1 : Sum  Inputs=+-  OutDataTypeStr=Inherit: Same as first input
  Compare To Constant : simulink/Logic and Bit Operations/Compare To Constant  relop=>=  const=4  OutDataTypeStr=boolean
  Complex to Real-Imag : ComplexToRealImag
  Constant : Constant  OutDataTypeStr=uint8  SampleTime=-1
  Data Type Conversion2 : DataTypeConversion
  Gain : Gain  Gain=2  OutDataTypeStr=Inherit: Same as input  ParamDataTypeStr=Inherit: Same as input
  Logical Operator : Logic  Operator=OR  IconShape=distinctive  AllPortsSameDT=off  OutDataTypeStr=boolean
  Product1 : Product
  Product2 : Product
  Product3 : Product
  Real-Imag to Complex : RealImagToComplex
  Sum : Sum  Inputs=|++  OutDataTypeStr=Inherit: Same as first input
  Sum1 : Sum  Inputs=|++
  Switch : Switch  Criteria=u2 ~= 0
  stop_out : Outport  VectorParamsAs1DForOutWhenUnconnected=off
  z_out : Outport  Port=2  VectorParamsAs1DForOutWhenUnconnected=off
  c_out : Outport  Port=3  VectorParamsAs1DForOutWhenUnconnected=off
  i_out : Outport  Port=4  VectorParamsAs1DForOutWhenUnconnected=off
  wires:
  i_in/1 -> Switch/1, Sum1/1
  c_in/1 -> c_out/1, Sum/2
  z_in/1 -> Complex to Real-Imag/1
  stop_in/1 -> Logical Operator/1
  Add/1 -> Compare To Constant/1
  Add1/1 -> Real-Imag to Complex/1
  Compare To Constant/1 -> Logical Operator/2
  Complex to Real-Imag/2 -> Product3/2, Product2/1, Product2/2
  Complex to Real-Imag/1 -> Product3/1, Product1/1, Product1/2
  Constant/1 -> Sum1/2
  Data Type Conversion2/1 -> z_out/1
  Gain/1 -> Real-Imag to Complex/2
  Logical Operator/1 -> stop_out/1, Switch/2
  Product1/1 -> Add1/1, Add/1
  Product2/1 -> Add1/2, Add/2
  Product3/1 -> Gain/1
  Real-Imag to Complex/1 -> Sum/1
  Sum/1 -> Data Type Conversion2/1
  Sum1/1 -> Switch/3
  Switch/1 -> i_out/1

== system gm_mandelbrot_fpga/mandelbrot_top/mandelbrot_core/mandelbroot_pipeline/mandelbroot_array_instance113 ==
  stop_in : Inport  OutDataTypeStr=boolean  PortDimensions=1  SampleTime=1.35e-08
  z_in : Inport  Port=2  OutDataTypeStr=fixdt(1, 18, 15)  PortDimensions=1  SampleTime=1.35e-08
      settings: SignalType=complex
  c_in : Inport  Port=3  OutDataTypeStr=fixdt(1, 18, 15)  PortDimensions=1  SampleTime=1.35e-08
      settings: SignalType=complex
  i_in : Inport  Port=4  OutDataTypeStr=fixdt(0, 7, 0)  PortDimensions=1  SampleTime=1.35e-08
  Add : Sum
  Add1 : Sum  Inputs=+-  OutDataTypeStr=Inherit: Same as first input
  Compare To Constant : simulink/Logic and Bit Operations/Compare To Constant  relop=>=  const=4  OutDataTypeStr=boolean
  Complex to Real-Imag : ComplexToRealImag
  Constant : Constant  OutDataTypeStr=uint8  SampleTime=-1
  Data Type Conversion2 : DataTypeConversion
  Gain : Gain  Gain=2  OutDataTypeStr=Inherit: Same as input  ParamDataTypeStr=Inherit: Same as input
  Logical Operator : Logic  Operator=OR  IconShape=distinctive  AllPortsSameDT=off  OutDataTypeStr=boolean
  Product1 : Product
  Product2 : Product
  Product3 : Product
  Real-Imag to Complex : RealImagToComplex
  Sum : Sum  Inputs=|++  OutDataTypeStr=Inherit: Same as first input
  Sum1 : Sum  Inputs=|++
  Switch : Switch  Criteria=u2 ~= 0
  stop_out : Outport  VectorParamsAs1DForOutWhenUnconnected=off
  z_out : Outport  Port=2  VectorParamsAs1DForOutWhenUnconnected=off
  c_out : Outport  Port=3  VectorParamsAs1DForOutWhenUnconnected=off
  i_out : Outport  Port=4  VectorParamsAs1DForOutWhenUnconnected=off
  wires:
  i_in/1 -> Switch/1, Sum1/1
  c_in/1 -> c_out/1, Sum/2
  z_in/1 -> Complex to Real-Imag/1
  stop_in/1 -> Logical Operator/1
  Add/1 -> Compare To Constant/1
  Add1/1 -> Real-Imag to Complex/1
  Compare To Constant/1 -> Logical Operator/2
  Complex to Real-Imag/2 -> Product3/2, Product2/1, Product2/2
  Complex to Real-Imag/1 -> Product3/1, Product1/1, Product1/2
  Constant/1 -> Sum1/2
  Data Type Conversion2/1 -> z_out/1
  Gain/1 -> Real-Imag to Complex/2
  Logical Operator/1 -> stop_out/1, Switch/2
  Product1/1 -> Add1/1, Add/1
  Product2/1 -> Add1/2, Add/2
  Product3/1 -> Gain/1
  Real-Imag to Complex/1 -> Sum/1
  Sum/1 -> Data Type Conversion2/1
  Sum1/1 -> Switch/3
  Switch/1 -> i_out/1

== system gm_mandelbrot_fpga/mandelbrot_top/mandelbrot_core/mandelbroot_pipeline/mandelbroot_array_instance114 ==
  stop_in : Inport  OutDataTypeStr=boolean  PortDimensions=1  SampleTime=1.35e-08
  z_in : Inport  Port=2  OutDataTypeStr=fixdt(1, 18, 15)  PortDimensions=1  SampleTime=1.35e-08
      settings: SignalType=complex
  c_in : Inport  Port=3  OutDataTypeStr=fixdt(1, 18, 15)  PortDimensions=1  SampleTime=1.35e-08
      settings: SignalType=complex
  i_in : Inport  Port=4  OutDataTypeStr=fixdt(0, 7, 0)  PortDimensions=1  SampleTime=1.35e-08
  Add : Sum
  Add1 : Sum  Inputs=+-  OutDataTypeStr=Inherit: Same as first input
  Compare To Constant : simulink/Logic and Bit Operations/Compare To Constant  relop=>=  const=4  OutDataTypeStr=boolean
  Complex to Real-Imag : ComplexToRealImag
  Constant : Constant  OutDataTypeStr=uint8  SampleTime=-1
  Data Type Conversion2 : DataTypeConversion
  Gain : Gain  Gain=2  OutDataTypeStr=Inherit: Same as input  ParamDataTypeStr=Inherit: Same as input
  Logical Operator : Logic  Operator=OR  IconShape=distinctive  AllPortsSameDT=off  OutDataTypeStr=boolean
  Product1 : Product
  Product2 : Product
  Product3 : Product
  Real-Imag to Complex : RealImagToComplex
  Sum : Sum  Inputs=|++  OutDataTypeStr=Inherit: Same as first input
  Sum1 : Sum  Inputs=|++
  Switch : Switch  Criteria=u2 ~= 0
  stop_out : Outport  VectorParamsAs1DForOutWhenUnconnected=off
  z_out : Outport  Port=2  VectorParamsAs1DForOutWhenUnconnected=off
  c_out : Outport  Port=3  VectorParamsAs1DForOutWhenUnconnected=off
  i_out : Outport  Port=4  VectorParamsAs1DForOutWhenUnconnected=off
  wires:
  i_in/1 -> Switch/1, Sum1/1
  c_in/1 -> c_out/1, Sum/2
  z_in/1 -> Complex to Real-Imag/1
  stop_in/1 -> Logical Operator/1
  Add/1 -> Compare To Constant/1
  Add1/1 -> Real-Imag to Complex/1
  Compare To Constant/1 -> Logical Operator/2
  Complex to Real-Imag/2 -> Product3/2, Product2/1, Product2/2
  Complex to Real-Imag/1 -> Product3/1, Product1/1, Product1/2
  Constant/1 -> Sum1/2
  Data Type Conversion2/1 -> z_out/1
  Gain/1 -> Real-Imag to Complex/2
  Logical Operator/1 -> stop_out/1, Switch/2
  Product1/1 -> Add1/1, Add/1
  Product2/1 -> Add1/2, Add/2
  Product3/1 -> Gain/1
  Real-Imag to Complex/1 -> Sum/1
  Sum/1 -> Data Type Conversion2/1
  Sum1/1 -> Switch/3
  Switch/1 -> i_out/1
